simulink model "PID_Controller"  (R2023b)
settings: Solver=VariableStepAuto  StartTime=0.0  StopTime=2  RelTol=1e-3
libraries: fl_lib x41, nesl_utility x8, ee_lib x2, simulink x1
settings Model: Creator=vkjk4  LastModifiedBy=vkjk4

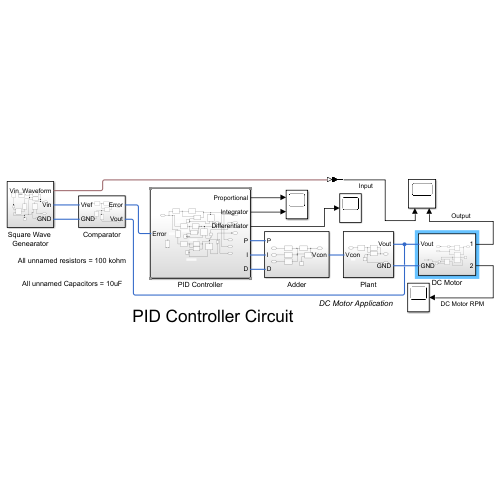
[thumbnail: Simulink's stored preview of the top-level diagram]
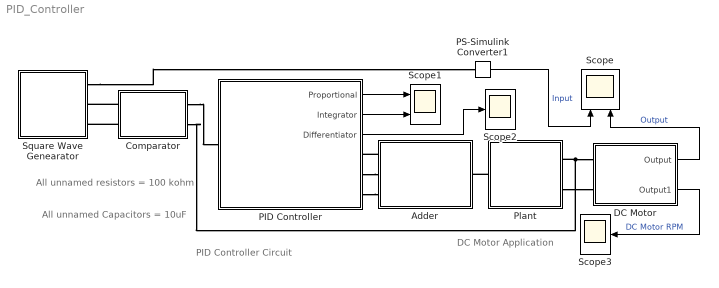
== system PID_Controller ==
  note: DC Motor Application
  note: All unnamed Capacitors = 10uF
  note: All unnamed resistors = 100 kohm
  note: PID Controller Circuit
  Adder : Subsystem
  Comparator : Subsystem
  DC Motor : Subsystem
  PID Controller : Subsystem
  PS-Simulink Converter1 : nesl_utility/PS-Simulink Converter  PhysicalDomain=network_engine_domain  SubClassName=ps_output  LeftPortType=input  RightPortType=output  PseudoPeriodic=off  Frequencies=[]  VectorFormat=inherit  Unit=inherit  AffineConversion=off
  Plant : Subsystem
  Scope : Scope  NumInputPorts=2
  Scope1 : Scope  NumInputPorts=2
  Scope2 : Scope
  Scope3 : Scope
  Square Wave Genearator : Subsystem
  wires:
  PS-Simulink Converter1/1 -> Scope/1  "Input"
  DC Motor/1(Output) -> Scope/2  "Output"
  DC Motor/2(Output1) -> Scope3/1  "DC Motor RPM"
  PID Controller/3(Differentiator) -> Scope2/1
  PID Controller/1(Proportional) -> Scope1/1
  PID Controller/2(Integrator) -> Scope1/2
  connections:
  Adder/LConn1 -- PID Controller/RConn1
  PID Controller/RConn2 -- Adder/LConn2
  PID Controller/RConn3 -- Adder/LConn3
  Plant/LConn1 -- Adder/RConn1
  Comparator/RConn1 -- PID Controller/LConn1
  Comparator/RConn2 -- Plant/RConn1 -- DC Motor/LConn1
  Plant/RConn2 -- DC Motor/LConn2
  Square Wave Genearator/RConn1 -- PS-Simulink Converter1/LConn1
  Comparator/LConn1 -- Square Wave Genearator/RConn2
  Comparator/LConn2 -- Square Wave Genearator/RConn3

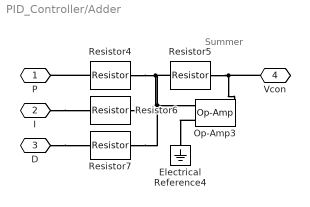
== system PID_Controller/Adder ==
  note: Summer
  Electrical Reference4 : fl_lib/Electrical/Electrical Elements/Electrical Reference
  Op-Amp3 : fl_lib/Electrical/Electrical Elements/Op-Amp  outI_specify=off  outI_priority=None  outI=0 A  outI_nominal_specify=off  outI_nominal_unit=A  outI_nominal_value=1
  Resistor4 : fl_lib/Electrical/Electrical Elements/Resistor  R=100 kOhm  i_specify=off  i_priority=None  i=0 A  i_nominal_specify=off  i_nominal_unit=A  i_nominal_value=1  v_specify=off  v_priority=None  v=0 V  v_nominal_specify=off  v_nominal_unit=V  v_nominal_value=1
  Resistor5 : fl_lib/Electrical/Electrical Elements/Resistor  R=100 kOhm  i_specify=off  i_priority=None  i=0 A  i_nominal_specify=off  i_nominal_unit=A  i_nominal_value=1  v_specify=off  v_priority=None  v=0 V  v_nominal_specify=off  v_nominal_unit=V  v_nominal_value=1
  Resistor6 : fl_lib/Electrical/Electrical Elements/Resistor  R=100 Ohm  i_specify=off  i_priority=None  i=0 A  i_nominal_specify=off  i_nominal_unit=A  i_nominal_value=1  v_specify=off  v_priority=None  v=0 V  v_nominal_specify=off  v_nominal_unit=V  v_nominal_value=1
  Resistor7 : fl_lib/Electrical/Electrical Elements/Resistor  R=100 kOhm  i_specify=off  i_priority=None  i=0 A  i_nominal_specify=off  i_nominal_unit=A  i_nominal_value=1  v_specify=off  v_priority=None  v=0 V  v_nominal_specify=off  v_nominal_unit=V  v_nominal_value=1
  P : PMIOPort  Side=Left
  I : PMIOPort  Port=2  Side=Left
  D : PMIOPort  Port=3  Side=Left
  Vcon : PMIOPort  Port=4  Side=Right
  connections:
  I/RConn1 -- Resistor6/LConn1
  Resistor4/RConn1 -- Resistor6/RConn1 -- Resistor7/RConn1 -- Op-Amp3/LConn2 -- Resistor5/LConn1
  Resistor5/RConn1 -- Vcon/RConn1 -- Op-Amp3/RConn1
  Op-Amp3/LConn1 -- Electrical Reference4/LConn1
  Resistor4/LConn1 -- P/RConn1
  D/RConn1 -- Resistor7/LConn1

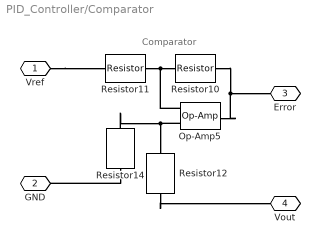
== system PID_Controller/Comparator ==
  note: Comparator
  Op-Amp5 : fl_lib/Electrical/Electrical Elements/Op-Amp  outI_specify=off  outI_priority=None  outI=0 A  outI_nominal_specify=off  outI_nominal_unit=A  outI_nominal_value=1
  Resistor{10..12,14} (4 alike) : fl_lib/Electrical/Electrical Elements/Resistor  R=100 kOhm  i_specify=off  i_priority=None  i=0 A  i_nominal_specify=off  i_nominal_unit=A  i_nominal_value=1  v_specify=off  v_priority=None  v=0 V  v_nominal_specify=off  v_nominal_unit=V  v_nominal_value=1
  Vref : PMIOPort  Side=Left
  GND : PMIOPort  Port=2  Side=Left
  Error : PMIOPort  Port=3  Side=Right
  Vout : PMIOPort  Port=4  Side=Right
  connections:
  Resistor10/RConn1 -- Error/RConn1 -- Op-Amp5/RConn1
  Vref/RConn1 -- Resistor11/LConn1
  Resistor11/RConn1 -- Op-Amp5/LConn2 -- Resistor10/LConn1
  Op-Amp5/LConn1 -- Resistor14/LConn1 -- Resistor12/LConn1
  Resistor12/RConn1 -- Vout/RConn1
  Resistor14/RConn1 -- GND/RConn1

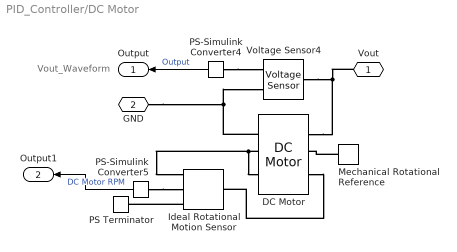
== system PID_Controller/DC Motor ==
  note: Vout_Waveform
  DC Motor : ee_lib/Electromechanical/Brushed Motors/DC Motor  Tag={'toolbox/physmod/elec/library/m/ee_lib_parts';'Electromechanical/Brushed_Motors/DC_Motor/AMETEK/DC040A_2.xml'}  field_option=ee.enum.field_option.pm  Rf=100 % Parameter not set Ohm  Lf=1 % Parameter not set H  Laf=0.15 % Parameter not set H  If0=0 % Parameter not set A  parameterization=ee.enum.dcparam_option.circuit_param  Ra=8.33 Ohm  La=6.17 mH  emf_or_torque=ee.enum.emf_or_torque.kv  Kv=4.14 mV/rpm  Ki=39.53409 % Parameter estimated mN*m/A  T_stall=0.24e-3 % Parameter not set N*m  w_max=19100 % Parameter not set rpm  w_rated=15000 % Parameter not set rpm  P_rated=0.08 % Parameter not set W  V_rated=1.5 % Parameter not set V  lam_param=ee.enum.lam_param.current  i_noload=0.14 A  V_i_noload=24 V  J=27.54 g*cm^2  lam=0 % % Parameter not set mN*m/(rad/s)  speed0=0 % Parameter not set rpm  enable_fault_armature=simscape.enum.onoff.off  rev_faulted=1 / 3 % Parameter not set  G_faulted_armature=1e-5 % Parameter not set S  fault_trigger_armature=ee.enum.faults.faultTrigger.temporal  t_fault_armature=1 % Parameter not set s  max_permissible_current_armature=inf % Parameter not set A  t_fail_on_current_armature=1 % Parameter not set s  enable_fault_field=simscape.enum.onoff.off  G_faulted_field=1e-5 % Parameter not set S  fault_trigger_field=ee.enum.faults.faultTrigger.temporal  t_fault_field=1 % Parameter not set s  max_permissible_current_field=inf % Parameter not set A  t_fail_on_current_field=1 % Parameter not set s  fault_action=simscape.enum.assert.action.none  alpha=3.93e-3 % Parameter not set 1/K  Tmeas=25 % Parameter not set degC  thermal_mass=88 % Parameter assumed J/K  initial_temperature=25 % Parameter not set degC
      settings: AttributesFormatString=AMETEK:DC040A_2
  Ideal Rotational Motion Sensor : fl_lib/Mechanical/Mechanical Sensors/Ideal Rotational Motion Sensor  reference=foundation.enum.MeasurementReference.difference  acceleration_port=false  velocity_port=true  position_port=true  wrap_angle=false  offset=0 rad
  Mechanical Rotational Reference : fl_lib/Mechanical/Rotational Elements/Mechanical Rotational Reference
  PS Terminator : fl_lib/Physical Signals/Sinks/PS Terminator
  PS-Simulink Converter4 : nesl_utility/PS-Simulink Converter  PhysicalDomain=network_engine_domain  SubClassName=ps_output  LeftPortType=input  RightPortType=output  PseudoPeriodic=off  Frequencies=[]  VectorFormat=inherit  Unit=inherit  AffineConversion=off
  PS-Simulink Converter5 : nesl_utility/PS-Simulink Converter  PhysicalDomain=network_engine_domain  SubClassName=ps_output  LeftPortType=input  RightPortType=output  PseudoPeriodic=off  Frequencies=[]  VectorFormat=inherit  Unit=inherit  AffineConversion=off
  Voltage Sensor4 : fl_lib/Electrical/Electrical Sensors/Voltage Sensor
  Vout : PMIOPort  Side=Left
  GND : PMIOPort  Port=2  Side=Left
  Output : Outport
  Output1 : Outport  Port=2
  wires:
  PS-Simulink Converter5/1 -> Output1/1  "DC Motor RPM"
  PS-Simulink Converter4/1 -> Output/1  "Output"
  connections:
  PS-Simulink Converter5/LConn1 -- Ideal Rotational Motion Sensor/RConn2
  PS-Simulink Converter4/LConn1 -- Voltage Sensor4/RConn1
  Ideal Rotational Motion Sensor/RConn3 -- PS Terminator/LConn1
  Mechanical Rotational Reference/LConn1 -- DC Motor/RConn2 -- Ideal Rotational Motion Sensor/RConn1
  Voltage Sensor4/LConn1 -- DC Motor/LConn1 -- Vout/RConn1
  DC Motor/RConn1 -- GND/RConn1 -- Voltage Sensor4/RConn2
  DC Motor/LConn2 -- Ideal Rotational Motion Sensor/LConn1

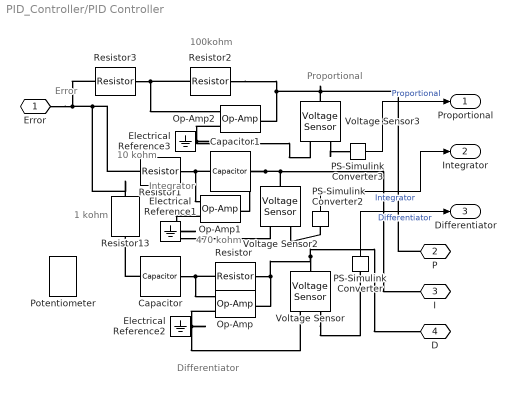
== system PID_Controller/PID Controller ==
  note: 470 kohm
  note: 1 kohm
  note: 10 kohm
  note: Differentiator
  note: Integrator
  note: Proportional
  note: Error
  note: 100kohm
  Capacitor : fl_lib/Electrical/Electrical Elements/Capacitor  c=10e-6 F  r=1e-6 Ohm  g=0 1/Ohm  i_specify=off  i_priority=None  i=0 A  i_nominal_specify=off  i_nominal_unit=A  i_nominal_value=1  v_specify=off  v_priority=None  v=0 V  v_nominal_specify=off  v_nominal_unit=V  v_nominal_value=1  vc_specify=off  vc_priority=High  vc=0 V  vc_nominal_specify=off  vc_nominal_unit=V  vc_nominal_value=1
  Capacitor1 : fl_lib/Electrical/Electrical Elements/Capacitor  c=10e-6 F  r=1e-6 Ohm  g=0 1/Ohm  i_specify=off  i_priority=None  i=0 A  i_nominal_specify=off  i_nominal_unit=A  i_nominal_value=1  v_specify=off  v_priority=None  v=0 V  v_nominal_specify=off  v_nominal_unit=V  v_nominal_value=1  vc_specify=off  vc_priority=High  vc=0 V  vc_nominal_specify=off  vc_nominal_unit=V  vc_nominal_value=1
  Electrical Reference1 : fl_lib/Electrical/Electrical Elements/Electrical Reference
  Electrical Reference2 : fl_lib/Electrical/Electrical Elements/Electrical Reference
  Electrical Reference3 : fl_lib/Electrical/Electrical Elements/Electrical Reference
  Op-Amp : fl_lib/Electrical/Electrical Elements/Op-Amp  outI_specify=off  outI_priority=None  outI=0 A  outI_nominal_specify=off  outI_nominal_unit=A  outI_nominal_value=1
  Op-Amp1 : fl_lib/Electrical/Electrical Elements/Op-Amp  outI_specify=off  outI_priority=None  outI=0 A  outI_nominal_specify=off  outI_nominal_unit=A  outI_nominal_value=1
  Op-Amp2 : fl_lib/Electrical/Electrical Elements/Op-Amp  outI_specify=off  outI_priority=None  outI=0 A  outI_nominal_specify=off  outI_nominal_unit=A  outI_nominal_value=1
  PS-Simulink Converter : nesl_utility/PS-Simulink Converter  PhysicalDomain=network_engine_domain  SubClassName=ps_output  LeftPortType=input  RightPortType=output  PseudoPeriodic=off  Frequencies=[]  VectorFormat=inherit  Unit=inherit  AffineConversion=off
  PS-Simulink Converter2 : nesl_utility/PS-Simulink Converter  PhysicalDomain=network_engine_domain  SubClassName=ps_output  LeftPortType=input  RightPortType=output  PseudoPeriodic=off  Frequencies=[]  VectorFormat=inherit  Unit=inherit  AffineConversion=off
  PS-Simulink Converter3 : nesl_utility/PS-Simulink Converter  PhysicalDomain=network_engine_domain  SubClassName=ps_output  LeftPortType=input  RightPortType=output  PseudoPeriodic=off  Frequencies=[]  VectorFormat=inherit  Unit=inherit  AffineConversion=off
  Potentiometer : ee_lib/Passive/Potentiometer  nPorts=ee.enum.passive.potentiometer.nPorts.Two  R0=200 kOhm  Rw=1 Ohm  xmin=0  xmax=1  minResistance=1 Ohm  maxResistance=1 MOhm  xmin2port=0  xmax2port=1  Taper=ee.enum.passive.potentiometer.linOrLog.lin  Rcenter=200 Ohm  Gradient=ee.enum.passive.potentiometer.gradient.higherR
      settings: InternalSimscapePortConfiguration="{\"Bottom\":[],\"Left\":[{\"id\":\"pinL\",\"label\":\"L\",\"type\":\"foundation.electrical.electrical\"},{\"id\":\"W\",\"label\":\"W\",\"type\":\"foundation.electrical.electrical\"}],\"Right\":[{\"id\":\"x\",\"label\":\"x\",\"type\":\"input\"}],\"Top\":[]}"
  Resistor : fl_lib/Electrical/Electrical Elements/Resistor  R=470 kOhm  i_specify=off  i_priority=None  i=0 A  i_nominal_specify=off  i_nominal_unit=A  i_nominal_value=1  v_specify=off  v_priority=None  v=0 V  v_nominal_specify=off  v_nominal_unit=V  v_nominal_value=1
  Resistor1 : fl_lib/Electrical/Electrical Elements/Resistor  R=10 kOhm  i_specify=off  i_priority=None  i=0 A  i_nominal_specify=off  i_nominal_unit=A  i_nominal_value=1  v_specify=off  v_priority=None  v=0 V  v_nominal_specify=off  v_nominal_unit=V  v_nominal_value=1
  Resistor13 : fl_lib/Electrical/Electrical Elements/Resistor  R=1 kOhm  i_specify=off  i_priority=None  i=0 A  i_nominal_specify=off  i_nominal_unit=A  i_nominal_value=1  v_specify=off  v_priority=None  v=0 V  v_nominal_specify=off  v_nominal_unit=V  v_nominal_value=1
  Resistor2 : fl_lib/Electrical/Electrical Elements/Resistor  R=100 kOhm  i_specify=off  i_priority=None  i=0 A  i_nominal_specify=off  i_nominal_unit=A  i_nominal_value=1  v_specify=off  v_priority=None  v=0 V  v_nominal_specify=off  v_nominal_unit=V  v_nominal_value=1
  Resistor3 : fl_lib/Electrical/Electrical Elements/Resistor  R=100 kOhm  i_specify=off  i_priority=None  i=0 A  i_nominal_specify=off  i_nominal_unit=A  i_nominal_value=1  v_specify=off  v_priority=None  v=0 V  v_nominal_specify=off  v_nominal_unit=V  v_nominal_value=1
  Voltage Sensor : fl_lib/Electrical/Electrical Sensors/Voltage Sensor
  Voltage Sensor2 : fl_lib/Electrical/Electrical Sensors/Voltage Sensor
  Voltage Sensor3 : fl_lib/Electrical/Electrical Sensors/Voltage Sensor
  Error : PMIOPort  Side=Left
  P : PMIOPort  Port=2  Side=Right
  I : PMIOPort  Port=3  Side=Right
  D : PMIOPort  Port=4  Side=Right
  Proportional : Outport
  Integrator : Outport  Port=2
  Differentiator : Outport  Port=3
  wires:
  PS-Simulink Converter3/1 -> Proportional/1  "Proportional"
  PS-Simulink Converter2/1 -> Integrator/1  "Integrator"
  PS-Simulink Converter/1 -> Differentiator/1  "Differentiator"
  connections:
  Capacitor/LConn1 -- Resistor13/RConn1
  Op-Amp1/LConn1 -- Electrical Reference1/LConn1 -- Voltage Sensor2/RConn2
  Resistor3/RConn1 -- Resistor2/LConn1 -- Op-Amp2/LConn2
  Capacitor/RConn1 -- Resistor/LConn1 -- Op-Amp/LConn2
  Voltage Sensor2/LConn1 -- I/RConn1 -- Capacitor1/RConn1 -- Op-Amp1/RConn1
  Resistor/RConn1 -- D/RConn1 -- Voltage Sensor/LConn1 -- Op-Amp/RConn1
  Op-Amp2/LConn1 -- Electrical Reference3/LConn1 -- Voltage Sensor3/RConn2
  Resistor1/LConn1 -- Resistor3/LConn1 -- Error/RConn1 -- Resistor13/LConn1
  Op-Amp/LConn1 -- Electrical Reference2/LConn1 -- Voltage Sensor/RConn2
  Voltage Sensor3/LConn1 -- P/RConn1 -- Resistor2/RConn1 -- Op-Amp2/RConn1
  Voltage Sensor3/RConn1 -- PS-Simulink Converter3/LConn1
  Capacitor1/LConn1 -- Resistor1/RConn1 -- Op-Amp1/LConn2
  Voltage Sensor2/RConn1 -- PS-Simulink Converter2/LConn1
  Voltage Sensor/RConn1 -- PS-Simulink Converter/LConn1

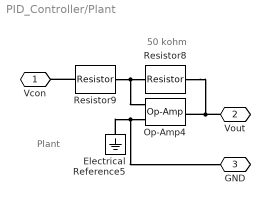
== system PID_Controller/Plant ==
  note: 50 kohm
  note: Plant
  Electrical Reference5 : fl_lib/Electrical/Electrical Elements/Electrical Reference
  Op-Amp4 : fl_lib/Electrical/Electrical Elements/Op-Amp  outI_specify=off  outI_priority=None  outI=0 A  outI_nominal_specify=off  outI_nominal_unit=A  outI_nominal_value=1
  Resistor8 : fl_lib/Electrical/Electrical Elements/Resistor  R=50 kOhm  i_specify=off  i_priority=None  i=0 A  i_nominal_specify=off  i_nominal_unit=A  i_nominal_value=1  v_specify=off  v_priority=None  v=0 V  v_nominal_specify=off  v_nominal_unit=V  v_nominal_value=1
  Resistor9 : fl_lib/Electrical/Electrical Elements/Resistor  R=100 kOhm  i_specify=off  i_priority=None  i=0 A  i_nominal_specify=off  i_nominal_unit=A  i_nominal_value=1  v_specify=off  v_priority=None  v=0 V  v_nominal_specify=off  v_nominal_unit=V  v_nominal_value=1
  Vcon : PMIOPort  Side=Left
  Vout : PMIOPort  Port=2  Side=Right
  GND : PMIOPort  Port=3  Side=Right
  connections:
  Resistor9/LConn1 -- Vcon/RConn1
  Electrical Reference5/LConn1 -- GND/RConn1 -- Op-Amp4/LConn1
  Resistor9/RConn1 -- Op-Amp4/LConn2 -- Resistor8/LConn1
  Vout/RConn1 -- Resistor8/RConn1 -- Op-Amp4/RConn1

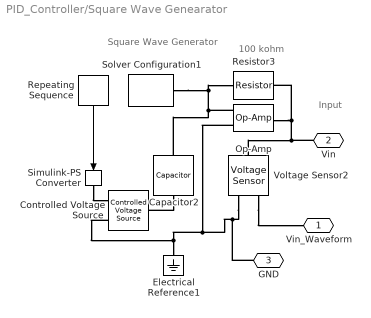
== system PID_Controller/Square Wave Genearator ==
  note: Square Wave Generator
  note: Input
  note: 100 kohm
  Capacitor2 : fl_lib/Electrical/Electrical Elements/Capacitor  c=10e-6 F  r=1e-6 Ohm  g=0 1/Ohm  i_specify=off  i_priority=None  i=0 A  i_nominal_specify=off  i_nominal_unit=A  i_nominal_value=1  v_specify=off  v_priority=None  v=0 V  v_nominal_specify=off  v_nominal_unit=V  v_nominal_value=1  vc_specify=off  vc_priority=High  vc=0 V  vc_nominal_specify=off  vc_nominal_unit=V  vc_nominal_value=1
  Controlled Voltage Source : fl_lib/Electrical/Electrical Sources/Controlled Voltage Source
  Electrical Reference1 : fl_lib/Electrical/Electrical Elements/Electrical Reference
  Op-Amp : fl_lib/Electrical/Electrical Elements/Op-Amp  outI_specify=off  outI_priority=None  outI=0 A  outI_nominal_specify=off  outI_nominal_unit=A  outI_nominal_value=1
  Repeating Sequence : simulink/Sources/Repeating Sequence  rep_seq_t=[0 0.5 1]  rep_seq_y=[0 1 0]
  Resistor3 : fl_lib/Electrical/Electrical Elements/Resistor  R=100 kOhm  i_specify=off  i_priority=None  i=0 A  i_nominal_specify=off  i_nominal_unit=A  i_nominal_value=1  v_specify=off  v_priority=None  v=0 V  v_nominal_specify=off  v_nominal_unit=V  v_nominal_value=1
  Simulink-PS Converter : nesl_utility/Simulink-PS Converter  PhysicalDomain=network_engine_domain  SubClassName=ps_input  LeftPortType=input  RightPortType=output  PseudoPeriodic=off  Frequencies=[]  NoiseDistribution=none  NoiseParameters=[]  Unit=1  AffineConversion=off  FilteringAndDerivatives=provide  SimscapeFilterOrder=1  InputFilterTimeConstant=0.001  UdotUserProvided=0
  Solver Configuration1 : nesl_utility/Solver Configuration  PhysicalDomain=network_engine_domain  SubClassName=solver  LeftPortType=input  RightPortType=generic  Tones=[]  Harmonics=[]  SimulateNoise=off  Profile=off  UseLocalSampling=off  EnableSwitchedLinearOptims=on  FrequencyDomain=off  UseCCode=off  RelTol=0.001  AbsTol=0.001  MinStep=1e-09  ToWorkspace=off  RevertToSquareIcSolve=off  NumHomotopyIterations=100  PhasorMode=off  PhasorModeNumHarmonics=1  ConsistencySolver=NEWTON_XTOL_AFTER_FTOL  IndexReductionMethod=DerivativeReplacement  DoDC=off  ResidualTolerance=1e-09  ConsistencyTolSource=GLOBAL  ConsistencyAbsTol=0.001  ConsistencyRelTol=0.001  ConsistencyTolFactor=0.001  UseLocalSolver=on  LocalSolverChoice=NE_BACKWARD_EULER_ADVANCER  ResolveIndetEquations=on  FunctionEvalNumThread=1  LocalSolverSampleTime=0.001  DoFixedCost=on  MaxNonlinIter=3  MaxModeIter=2  ComputeImpulses=off  ImpulseIterations=2  LinearAlgebra=auto  LinearAlgebraNumThread=0  EquationFormulation=NE_TIME_EF  DelaysMemoryBudget=1024  AutomaticFiltering=on  FilteringTimeConstant=0.001  PartitionStorageMethod=AS_NEEDED  PartitionMemoryBudget=1024  PartitionMethod=ROBUST  MultibodyUseLocalSolver=on  MultibodyLocalSolverChoice=ODE1  MultibodyLocalSolverSampleTime=0.001
  Voltage Sensor2 : fl_lib/Electrical/Electrical Sensors/Voltage Sensor
  Vin_Waveform : PMIOPort  Side=Right
  Vin : PMIOPort  Port=2  Side=Right
  GND : PMIOPort  Port=3  Side=Right
  wires:
  Repeating Sequence/1 -> Simulink-PS Converter/1
  connections:
  Vin/RConn1 -- Voltage Sensor2/LConn1 -- Op-Amp/RConn1 -- Resistor3/RConn1
  Voltage Sensor2/RConn1 -- Vin_Waveform/RConn1
  Capacitor2/LConn1 -- Controlled Voltage Source/LConn1
  Controlled Voltage Source/RConn2 -- Op-Amp/LConn1 -- Voltage Sensor2/RConn2 -- GND/RConn1 -- Electrical Reference1/LConn1
  Capacitor2/RConn1 -- Op-Amp/LConn2 -- Solver Configuration1/RConn1 -- Resistor3/LConn1
  Simulink-PS Converter/RConn1 -- Controlled Voltage Source/RConn1
